simulink model "piezoelectrico"  (R2020a)
settings: Solver=VariableStepAuto  StartTime=0.0  StopTime=10.0  RelTol=1e-3
undefined symbols (not defined in the file): den_anti, den_des, den_piezo, fs, g, num_anti, num_des, num_piezo, sens_piezo
libraries: simulink x1, simulink_extras x1
settings Model: Creator=Noxi-PC  LastModifiedBy=Noxi-PC

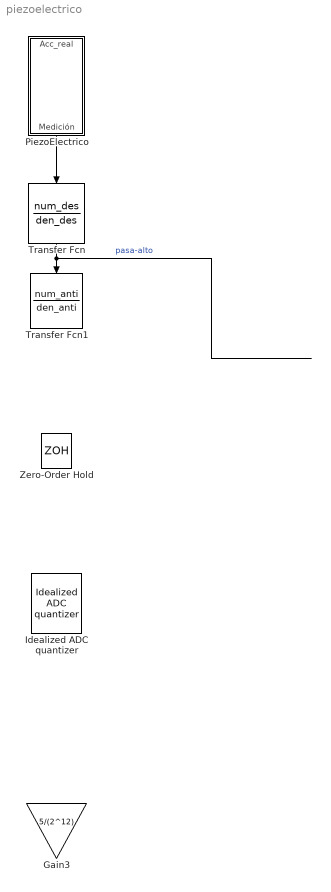
== system piezoelectrico ==
  " PiezoElectrico" : Subsystem
  Gain3 : Gain  Gain=5/(2^12)
  Idealized ADC quantizer : simulink_extras/Additional Discrete/Idealized ADC quantizer  NumberOfConverterBits=12  Vmin=-2.5  Vmax=2.5  OutputDataType=int16  OutputNegativeValues=on
  Transfer Fcn : TransferFcn  Numerator=num_des  Denominator=den_des
  Transfer Fcn1 : TransferFcn  Numerator=num_anti  Denominator=den_anti
  Zero-Order Hold : ZeroOrderHold  SampleTime=1/fs
  wires:
  ? -> " PiezoElectrico"/1(Acc_real)  "x2''"
  Transfer Fcn/1 -> Transfer Fcn1/1  "pasa-alto"
  " PiezoElectrico"/1(Medición) -> Transfer Fcn/1

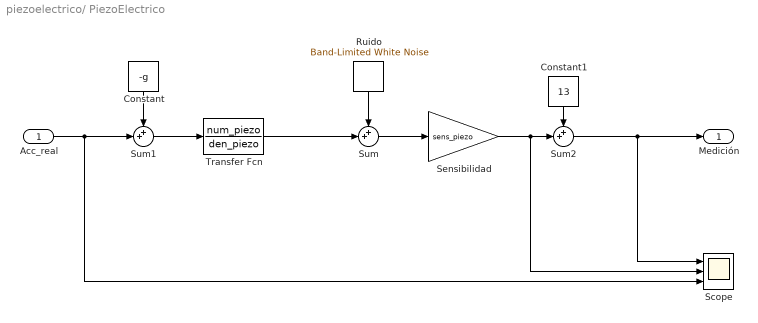
== system piezoelectrico/ PiezoElectrico ==
  Acc_real : Inport
  Constant : Constant  Value=-g
  Constant1 : Constant  Value=13
  Ruido : simulink/Sources/Band-Limited White Noise  Cov=NoisePower_piezo  Ts=1/fs  seed=[23341]
  Scope : Scope  NumInputPorts=3
  Sensibilidad : Gain  Gain=sens_piezo
  Sum : Sum  Inputs=++|
  Sum1 : Sum  Inputs=++|
  Sum2 : Sum  Inputs=++|
  Transfer Fcn : TransferFcn  Numerator=num_piezo  Denominator=den_piezo
  Medición : Outport
  wires:
  Transfer Fcn/1 -> Sum/2
  Ruido/1 -> Sum/1
  Constant/1 -> Sum1/1
  Sum1/1 -> Transfer Fcn/1
  Acc_real/1 -> Scope/3, Sum1/2
  Sum/1 -> Sensibilidad/1
  Constant1/1 -> Sum2/1
  Sensibilidad/1 -> Scope/2, Sum2/2
  Sum2/1 -> Medición/1, Scope/1
